simulink model "Examen_Sim4_v1"  (R2022a)
settings: Solver=VariableStepAuto  StartTime=0.0  StopTime=15  RelTol=1e-3
values from neighbouring files (symbols this model uses):
  A = [22 7 11;-64 -19 -26;-26 -8 -16]    [untitled2.m]
  B = [2;-4;-3]    [untitled2.m]
  K = cell(1,NoEqns)    [untitled2.m]
undefined symbols (not defined in the file or in its folder): C, D, L, t1, x0, x0b, Yeq
settings Model: Creator=fernando  LastModifiedBy=fernando

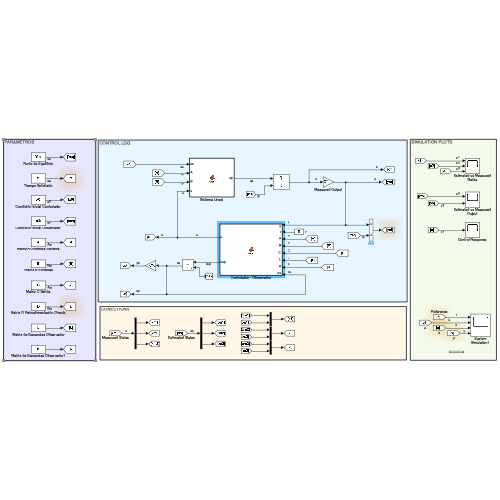
[thumbnail: Simulink's stored preview of the top-level diagram]
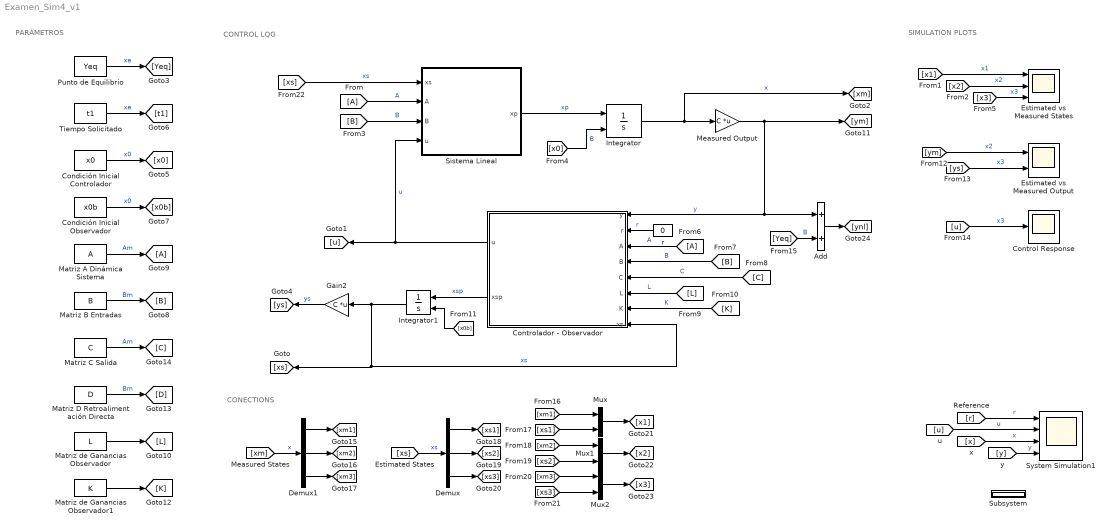
== system Examen_Sim4_v1 ==
  note: CONECTIONS
  note: CONTROL LQG
  note: SIMULATION PLOTS
  note: PARÁMETROS
  " Matriz B Entradas" : Constant  Value=B  VectorParams1D=off
  " Matriz de Ganancias Observador" : Constant  Value=L  VectorParams1D=off
  " Matriz de Ganancias Observador1" : Constant  Value=K  VectorParams1D=off
  Add : Sum
  Condición Inicial Controlador : Constant  Value=x0  VectorParams1D=off
  Condición Inicial Observador : Constant  Value=x0b  VectorParams1D=off
  Control Response : Scope
  Controlador - Observador : MATLAB Function  TreatAsAtomicUnit=on
  Demux : Demux  Outputs=3
  Demux1 : Demux  Outputs=3
  Estimated vs Measured Output : Scope  NumInputPorts=2
  Estimated vs Measured States : Scope  NumInputPorts=3
  From : From
  From6 : From
  Gain2 : Gain  Gain=C  Multiplication=Matrix(K*u)
  Goto9 : Goto
  Integrator : Integrator  InitialConditionSource=external  InitialCondition=x0
  Integrator1 : Integrator  InitialConditionSource=external  InitialCondition=x0b
  Matriz A Dinámica Sistema : Constant  Value=A  VectorParams1D=off
  Matriz C Salida : Constant  Value=C  VectorParams1D=off
  Matriz D Retroalimentación Directa : Constant  Value=D  VectorParams1D=off
  Measured Output : Gain  Gain=C  Multiplication=Matrix(K*u)
  Mux : Mux  Inputs=2
  Mux1 : Mux  Inputs=2
  Mux2 : Mux  Inputs=2
  Punto de Equilibrio : Constant  Value=Yeq  VectorParams1D=off
  Sistema Lineal : MATLAB Function  TreatAsAtomicUnit=on
  Subsystem : Subsystem
  System Simulation1 : Scope  NumInputPorts=4
  Tiempo Solicitado : Constant  Value=t1  VectorParams1D=off
  r : Constant  Value=0  VectorParams1D=off
  wires:
  Punto de Equilibrio/1 -> [Yeq]  "xe"
  Condición Inicial Observador/1 -> [x0b]  "x0"
  " Matriz B Entradas"/1 -> [B]  "Bm"
  Matriz A Dinámica Sistema/1 -> Goto9/1  "Am"
  " Matriz de Ganancias Observador"/1 -> [L]
  " Matriz de Ganancias Observador1"/1 -> [K]
  Matriz C Salida/1 -> [C]  "Am"
  Matriz D Retroalimentación Directa/1 -> [D]  "Bm"
  Condición Inicial Controlador/1 -> [x0]  "x0"
  Tiempo Solicitado/1 -> [t1]  "xe"
  [C] -> Controlador - Observador/5(C)  "C"
  Sistema Lineal/1(xp) -> Integrator/1  "xp"
  From6/1 -> Controlador - Observador/3(A)  "A"
  r/1 -> Controlador - Observador/2(r)  "r"
  Controlador - Observador/2(xsp) -> Integrator1/1  "xsp"
  [L] -> Controlador - Observador/6(L)  "L"
  Gain2/1 -> [ys]  "ys"
  Integrator1/1 -> Gain2/1, Controlador - Observador/8(xs), [xs]  "xs"
  Controlador - Observador/1(u) -> [u], Sistema Lineal/4(u)  "u"
  Measured Output/1 -> [ym], Controlador - Observador/1(y), Add/1  "y"
  Integrator/1 -> [xm], Measured Output/1  "x"
  [B] -> Sistema Lineal/3(B)  "B"
  [B] -> Controlador - Observador/4(B)  "B"
  [K] -> Controlador - Observador/7(K)  "K"
  From/1 -> Sistema Lineal/2(A)  "A"
  [x0] -> Integrator/2  "B"
  [x0b] -> Integrator1/2
  Demux/1 -> [xs1]
  Demux/2 -> [xs2]
  Demux1/2 -> [xm2]
  Demux/3 -> [xs3]
  Demux1/3 -> [xm3]
  Demux1/1 -> [xm1]
  [xm] -> Demux1/1  "x"
  [xs] -> Demux/1  "xs"
  [xm1] -> Mux/1
  [xs1] -> Mux/2
  [xs2] -> Mux1/2
  [xm3] -> Mux2/1
  [xm2] -> Mux1/1
  [xs3] -> Mux2/2
  Mux2/1 -> [x3]
  Mux/1 -> [x1]
  Mux1/1 -> [x2]
  [x3] -> Estimated vs Measured States/3  "x3"
  [x2] -> Estimated vs Measured States/2  "x2"
  [x1] -> Estimated vs Measured States/1  "x1"
  [ym] -> Estimated vs Measured Output/1  "x2"
  [ys] -> Estimated vs Measured Output/2  "x3"
  [u] -> Control Response/1  "x3"
  [r] -> System Simulation1/1  "r"
  [x] -> System Simulation1/3  "x"
  [u] -> System Simulation1/2  "u"
  [y] -> System Simulation1/4  "y"
  [Yeq] -> Add/2  "B"
  Add/1 -> [ynl]
  [xs] -> Sistema Lineal/1(xs)  "xs"

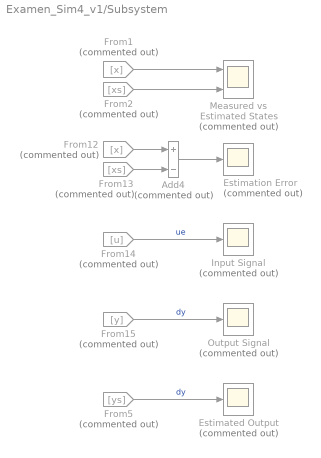
== system Examen_Sim4_v1/Subsystem ==
  Add4 : Sum  Commented=on  Inputs=+-
  Estimated Output : Scope  Commented=on
  Estimation Error : Scope  Commented=on
  From1 : From  Commented=on  GotoTag=x
  From12 : From  Commented=on  GotoTag=x
  From13 : From  Commented=on  GotoTag=xs
  From14 : From  Commented=on  GotoTag=u
  From15 : From  Commented=on  GotoTag=y
  From2 : From  Commented=on  GotoTag=xs
  From5 : From  Commented=on  GotoTag=ys
  Input Signal : Scope  Commented=on
  Measured vs Estimated States : Scope  Commented=on  NumInputPorts=2
  Output Signal : Scope  Commented=on
  wires:
  From5/1 -> Estimated Output/1  "dy"
  From13/1 -> Add4/2
  Add4/1 -> Estimation Error/1
  From15/1 -> Output Signal/1  "dy"
  From14/1 -> Input Signal/1  "ue"
  From12/1 -> Add4/1
  From1/1 -> Measured vs Estimated States/1
  From2/1 -> Measured vs Estimated States/2

== matlab function Examen_Sim4_v1/Sistema Lineal ==
  data: xs input; A input; B input; xp output; u input
function xp = fcn(xs,A,B,u)

xp = A*xs + B*u;

== matlab function Examen_Sim4_v1/Controlador - Observador ==
  data: y input; r input; A input; B input; C input; L input; K input; u output; xs input; xsp output
function [u,xsp] = fcn(y,r,A,B,C,L,K,xs)

xsp = (A - L*C - B*K)*(xs) + B*(r) + L*(y);

u = -K*xs + r;
